simulink model "SingleTrackCANoe"  (R2021b)
settings: Solver=ode1  StartTime=0  StopTime=2  FixedStep=1.0000000000000000e-003  RelTol=1e-3
InitFcn:
  | sampleTime = str2double(get_param(bdroot, 'FixedStep'));
undefined symbols (not defined in the file or in its folder): AccPedalPos, BrakePedalPos, BrakeSwitch, DiscIntNeverNeededParam, DYNA4, EngSpd, IgnitionSwitch, InitialGear, InitialSpeed, IntendedEngTrq, LeftIndicator, MainBrakePress, MaxGear, MDL, MinGear, RefAcc, RefLane, RefLatPos, RefPath, RefPathCurv, RefSpd, RefSpdPreview, RefSpdRetrospect, RightIndicator, SteeringWheelAng, SteeringWheelTrq, UserDefinedRefValue, vm_const
libraries: UtilitiesLibrary x62, simulink x18, WheelSystemModules x14, LongitudinalControllerModules x13, LateralControllerModules x7, AnimationBusselectorModules x5, EnvironmentModules x5, BasicEngineControlModules x5, MiscellaneousControlModules x5, Animation3Modules x4, AuxiliariesModules x4, ReducedTireModules x4
(part 28 of 34)

== system SingleTrackCANoe/SimulationModel/Vehicle/Drivetrain/DrivetrainPhysics/DrivetrainPhysicsInputs/InputFromDrivetrainControlUnit ==
  fromDrivetrainControlUnit : Inport
  TDBusSelector : BusSelector  OutputSignals=TransmissionControlUnit.Gear[-4;20],TransmissionControlUnit.AutomatedManualClutchPos[0_1]
  __TDD__AutomatedManualClutchPos[0_1] : Demux  Outputs=[1]
  __TDD__AutomaticGear[-4;20] : Demux  Outputs=[1]
  AutomaticGear[-4;20]___UNIQUE_1 : Outport  Description=|  PortDimensions=[1]  VectorParamsAs1DForOutWhenUnconnected=off
      | <name>TransmissionControlUnit.Gear[-4;20]</name>
      | <comment></comment>
  AutomatedManualClutchPos[0_1]___UNIQUE_1 : Outport  Description=|  Port=2  PortDimensions=[1]  VectorParamsAs1DForOutWhenUnconnected=off
      | <name>TransmissionControlUnit.AutomatedManualClutchPos[0_1]</name>
      | <comment></comment>
  wires:
  __TDD__AutomatedManualClutchPos[0_1]/1 -> AutomatedManualClutchPos[0_1]___UNIQUE_1/1  "AutomatedManualClutchPos[0_1]"
  __TDD__AutomaticGear[-4;20]/1 -> AutomaticGear[-4;20]___UNIQUE_1/1  "AutomaticGear[-4;20]"
  TDBusSelector/2 -> __TDD__AutomatedManualClutchPos[0_1]/1  "<AutomatedManualClutchPos[0_1]>"
  TDBusSelector/1 -> __TDD__AutomaticGear[-4;20]/1  "<Gear[-4;20]>"
  fromDrivetrainControlUnit/1 -> TDBusSelector/1

== system SingleTrackCANoe/SimulationModel/Vehicle/Drivetrain/DrivetrainPhysics/DrivetrainPhysicsInputs/InputFromEngine ==
  fromEngine : Inport
  TDBusSelector : BusSelector  OutputSignals=EnginePhysics.Mechanics.EngInrt[kg*m**2],EnginePhysics.Mechanics.EngTrq[Nm],EnginePhysics.Mechanics.DerivativeOfEngTrq_wrt_CrankAng[Nm/rad],EnginePhysics.Mechanics.DerivativeOfEngTrq_wrt_EngSpd[Nm/(rad/s)],EnginePhysics.Mechanics.MeanEngFrictionTrq[Nm],EngineControlUnit.EngIdleSpd[rad/s]
  __TDD__DerivativeOfEngTrq_wrt_CrankAng[Nm/rad] : Demux  Outputs=[1]
  __TDD__DerivativeOfEngTrq_wrt_EngSpd[Nm/(rad/s)] : Demux  Outputs=[1]
  __TDD__EngIdleSpd[rad/s] : Demux  Outputs=[1]
  __TDD__EngInrt[kg*m**2] : Demux  Outputs=[1]
  __TDD__EngTrq[Nm] : Demux  Outputs=[1]
  __TDD__MeanEngFrictionTrq[Nm] : Demux  Outputs=[1]
  EngInrt[kg*m**2]___UNIQUE_1 : Outport  Description=|  PortDimensions=[1]  VectorParamsAs1DForOutWhenUnconnected=off
      | <name>EnginePhysics.Mechanics.EngInrt[kg*m**2]</name>
      | <comment></comment>
  EngTrq[Nm]___UNIQUE_1 : Outport  Description=|  Port=2  PortDimensions=[1]  VectorParamsAs1DForOutWhenUnconnected=off
      | <name>EnginePhysics.Mechanics.EngTrq[Nm]</name>
      | <comment></comment>
  DerivativeOfEngTrq_wrt_CrankAng[Nm/rad]___UNIQUE_1 : Outport  Description=|  Port=3  PortDimensions=[1]  VectorParamsAs1DForOutWhenUnconnected=off
      | <name>EnginePhysics.Mechanics.DerivativeOfEngTrq_wrt_CrankAng[Nm/rad]</name>
      | <comment></comment>
  DerivativeOfEngTrq_wrt_EngSpd[Nm/(rad/s)]___UNIQUE_1 : Outport  Description=|  Port=4  PortDimensions=[1]  VectorParamsAs1DForOutWhenUnconnected=off
      | <name>EnginePhysics.Mechanics.DerivativeOfEngTrq_wrt_EngSpd[Nm/(rad/s)]</name>
      | <comment></comment>
  MeanEngFrictionTrq[Nm]___UNIQUE_1 : Outport  Description=|  Port=5  PortDimensions=[1]  VectorParamsAs1DForOutWhenUnconnected=off
      | <name>EnginePhysics.Mechanics.MeanEngFrictionTrq[Nm]</name>
      | <comment></comment>
  EngIdleSpd[rad/s]___UNIQUE_1 : Outport  Description=|  Port=6  PortDimensions=[1]  VectorParamsAs1DForOutWhenUnconnected=off
      | <name>EngineControlUnit.EngIdleSpd[rad/s]</name>
      | <comment></comment>
  wires:
  __TDD__EngIdleSpd[rad/s]/1 -> EngIdleSpd[rad/s]___UNIQUE_1/1  "EngIdleSpd[rad/s]"
  __TDD__MeanEngFrictionTrq[Nm]/1 -> MeanEngFrictionTrq[Nm]___UNIQUE_1/1  "MeanEngFrictionTrq[Nm]"
  __TDD__DerivativeOfEngTrq_wrt_EngSpd[Nm/(rad/s)]/1 -> DerivativeOfEngTrq_wrt_EngSpd[Nm/(rad/s)]___UNIQUE_1/1  "DerivativeOfEngTrq_wrt_EngSpd[Nm/(rad/s)]"
  __TDD__DerivativeOfEngTrq_wrt_CrankAng[Nm/rad]/1 -> DerivativeOfEngTrq_wrt_CrankAng[Nm/rad]___UNIQUE_1/1  "DerivativeOfEngTrq_wrt_CrankAng[Nm/rad]"
  __TDD__EngTrq[Nm]/1 -> EngTrq[Nm]___UNIQUE_1/1  "EngTrq[Nm]"
  __TDD__EngInrt[kg*m**2]/1 -> EngInrt[kg*m**2]___UNIQUE_1/1  "EngInrt[kg*m**2]"
  TDBusSelector/6 -> __TDD__EngIdleSpd[rad/s]/1  "<EngIdleSpd[rad/s]>"
  TDBusSelector/5 -> __TDD__MeanEngFrictionTrq[Nm]/1  "<MeanEngFrictionTrq[Nm]>"
  TDBusSelector/4 -> __TDD__DerivativeOfEngTrq_wrt_EngSpd[Nm/(rad/s)]/1  "<DerivativeOfEngTrq_wrt_EngSpd[Nm/(rad/s)]>"
  TDBusSelector/3 -> __TDD__DerivativeOfEngTrq_wrt_CrankAng[Nm/rad]/1  "<DerivativeOfEngTrq_wrt_CrankAng[Nm/rad]>"
  TDBusSelector/2 -> __TDD__EngTrq[Nm]/1  "<EngTrq[Nm]>"
  TDBusSelector/1 -> __TDD__EngInrt[kg*m**2]/1  "<EngInrt[kg*m**2]>"
  fromEngine/1 -> TDBusSelector/1

== system SingleTrackCANoe/SimulationModel/Vehicle/Drivetrain/DrivetrainPhysics/DrivetrainPhysicsInputs/InputFromWheelSystem ==
  fromWheelSystem : Inport
  TDBusSelector : BusSelector  OutputSignals=FrontLeft.Wheel.RotAcc[rad/s**2],FrontRight.Wheel.RotAcc[rad/s**2],RearLeft.Wheel.RotAcc[rad/s**2],RearRight.Wheel.RotAcc[rad/s**2],FrontLeft.Wheel.RotSpd[rad/s],FrontRight.Wheel.RotSpd[rad/s],RearLeft.Wheel.RotSpd[rad/s],RearRight.Wheel.RotSpd[rad/s],FrontLeft.Wheel.DriveBrakeTrq_wrt_WheelRotAxis(VehSys)[Nm],FrontRight.Wheel.DriveBrakeTrq_wrt_WheelRotAxis(VehSys)[Nm],RearLeft.Wheel.DriveBrakeTrq_wrt_WheelRotAxis(VehSys)[Nm],RearRight.Wheel.DriveBrakeTrq_wrt_WheelRotAxis(VehSys)[Nm],FrontLeft.Wheel.TotalResistanceTorque[Nm],FrontLeft.Wheel.RotAxisInrt[kg*m**2],FrontRight.Wheel.RotAxisInrt[kg*m**2],RearLeft.Wheel.RotAxisInrt[kg*m**2],RearRight.Wheel.RotAxisInrt[kg*m**2],FrontLeft.Wheel.VehBodyReplacementInrt[kg*m**2],FrontLeft.Wheel.KinematicWheelActiveFlag[0;1]
  __TDD__FrontLeft_Wheel_DriveBrakeTrq_wrt_WheelRotAxis(VehSys)[Nm] : Demux  Outputs=[3]
  __TDD__FrontLeft_Wheel_RotAcc[rad/s**2] : Demux  Outputs=1
  __TDD__FrontLeft_Wheel_RotAxisInrt[kg*m**2] : Demux  Outputs=[1]
  __TDD__FrontLeft_Wheel_RotSpd[rad/s] : Demux  Outputs=[1]
  __TDD__FrontRight_Wheel_DriveBrakeTrq_wrt_WheelRotAxis(VehSys)[Nm] : Demux  Outputs=[3]
  __TDD__FrontRight_Wheel_RotAcc[rad/s**2] : Demux  Outputs=1
  __TDD__FrontRight_Wheel_RotAxisInrt[kg*m**2] : Demux  Outputs=[1]
  __TDD__FrontRight_Wheel_RotSpd[rad/s] : Demux  Outputs=[1]
  __TDD__KinematicWheelActiveFlag[0;1] : Demux  Outputs=[1]
  __TDD__RearLeft_Wheel_DriveBrakeTrq_wrt_WheelRotAxis(VehSys)[Nm] : Demux  Outputs=[3]
  __TDD__RearLeft_Wheel_RotAcc[rad/s**2] : Demux  Outputs=1
  __TDD__RearLeft_Wheel_RotAxisInrt[kg*m**2] : Demux  Outputs=[1]
  __TDD__RearLeft_Wheel_RotSpd[rad/s] : Demux  Outputs=[1]
  __TDD__RearRight_Wheel_DriveBrakeTrq_wrt_WheelRotAxis(VehSys)[Nm] : Demux  Outputs=[3]
  __TDD__RearRight_Wheel_RotAcc[rad/s**2] : Demux  Outputs=1
  __TDD__RearRight_Wheel_RotAxisInrt[kg*m**2] : Demux  Outputs=[1]
  __TDD__RearRight_Wheel_RotSpd[rad/s] : Demux  Outputs=[1]
  __TDD__TotalResistanceTorque[Nm] : Demux  Outputs=[1]
  __TDD__VehBodyReplacementInrt[kg*m**2] : Demux  Outputs=[1]
  FrontLeft_Wheel_RotAcc[rad/s**2]___UNIQUE_1 : Outport  Description=|  VectorParamsAs1DForOutWhenUnconnected=off
      | <name>FrontLeft.Wheel.RotAcc[rad/s**2]</name>
      | <comment></comment>
  FrontRight_Wheel_RotAcc[rad/s**2]___UNIQUE_1 : Outport  Description=|  Port=2  VectorParamsAs1DForOutWhenUnconnected=off
      | <name>FrontRight.Wheel.RotAcc[rad/s**2]</name>
      | <comment></comment>
  RearLeft_Wheel_RotAcc[rad/s**2]___UNIQUE_1 : Outport  Description=|  Port=3  VectorParamsAs1DForOutWhenUnconnected=off
      | <name>RearLeft.Wheel.RotAcc[rad/s**2]</name>
      | <comment></comment>
  RearRight_Wheel_RotAcc[rad/s**2]___UNIQUE_1 : Outport  Description=|  Port=4  VectorParamsAs1DForOutWhenUnconnected=off
      | <name>RearRight.Wheel.RotAcc[rad/s**2]</name>
      | <comment></comment>
  FrontLeft_Wheel_RotSpd[rad/s]___UNIQUE_1 : Outport  Description=|  Port=5  PortDimensions=[1]  VectorParamsAs1DForOutWhenUnconnected=off
      | <name>FrontLeft.Wheel.RotSpd[rad/s]</name>
      | <comment></comment>
  FrontRight_Wheel_RotSpd[rad/s]___UNIQUE_1 : Outport  Description=|  Port=6  PortDimensions=[1]  VectorParamsAs1DForOutWhenUnconnected=off
      | <name>FrontRight.Wheel.RotSpd[rad/s]</name>
      | <comment></comment>
  RearLeft_Wheel_RotSpd[rad/s]___UNIQUE_1 : Outport  Description=|  Port=7  PortDimensions=[1]  VectorParamsAs1DForOutWhenUnconnected=off
      | <name>RearLeft.Wheel.RotSpd[rad/s]</name>
      | <comment></comment>
  RearRight_Wheel_RotSpd[rad/s]___UNIQUE_1 : Outport  Description=|  Port=8  PortDimensions=[1]  VectorParamsAs1DForOutWhenUnconnected=off
      | <name>RearRight.Wheel.RotSpd[rad/s]</name>
      | <comment></comment>
  FrontLeft_Wheel_DriveBrakeTrq_wrt_WheelRotAxis(VehSys)[Nm]___UNIQUE_1 : Outport  Description=|  Port=9  PortDimensions=[3]  VectorParamsAs1DForOutWhenUnconnected=off
      | <name>FrontLeft.Wheel.DriveBrakeTrq_wrt_WheelRotAxis(VehSys)[Nm]</name>
      | <comment></comment>
  FrontRight_Wheel_DriveBrakeTrq_wrt_WheelRotAxis(VehSys)[Nm]___UNIQUE_1 : Outport  Description=|  Port=10  PortDimensions=[3]  VectorParamsAs1DForOutWhenUnconnected=off
      | <name>FrontRight.Wheel.DriveBrakeTrq_wrt_WheelRotAxis(VehSys)[Nm]</name>
      | <comment></comment>
  RearLeft_Wheel_DriveBrakeTrq_wrt_WheelRotAxis(VehSys)[Nm]___UNIQUE_1 : Outport  Description=|  Port=11  PortDimensions=[3]  VectorParamsAs1DForOutWhenUnconnected=off
      | <name>RearLeft.Wheel.DriveBrakeTrq_wrt_WheelRotAxis(VehSys)[Nm]</name>
      | <comment></comment>
  RearRight_Wheel_DriveBrakeTrq_wrt_WheelRotAxis(VehSys)[Nm]___UNIQUE_1 : Outport  Description=|  Port=12  PortDimensions=[3]  VectorParamsAs1DForOutWhenUnconnected=off
      | <name>RearRight.Wheel.DriveBrakeTrq_wrt_WheelRotAxis(VehSys)[Nm]</name>
      | <comment></comment>
  TotalResistanceTorque[Nm]___UNIQUE_1 : Outport  Description=|  Port=13  PortDimensions=[1]  VectorParamsAs1DForOutWhenUnconnected=off
      | <name>FrontLeft.Wheel.TotalResistanceTorque[Nm]</name>
      | <comment></comment>
  FrontLeft_Wheel_RotAxisInrt[kg*m**2]___UNIQUE_1 : Outport  Description=|  Port=14  PortDimensions=[1]  VectorParamsAs1DForOutWhenUnconnected=off
      | <name>FrontLeft.Wheel.RotAxisInrt[kg*m**2]</name>
      | <comment></comment>
  FrontRight_Wheel_RotAxisInrt[kg*m**2]___UNIQUE_1 : Outport  Description=|  Port=15  PortDimensions=[1]  VectorParamsAs1DForOutWhenUnconnected=off
      | <name>FrontRight.Wheel.RotAxisInrt[kg*m**2]</name>
      | <comment></comment>
  RearLeft_Wheel_RotAxisInrt[kg*m**2]___UNIQUE_1 : Outport  Description=|  Port=16  PortDimensions=[1]  VectorParamsAs1DForOutWhenUnconnected=off
      | <name>RearLeft.Wheel.RotAxisInrt[kg*m**2]</name>
      | <comment></comment>
  RearRight_Wheel_RotAxisInrt[kg*m**2]___UNIQUE_1 : Outport  Description=|  Port=17  PortDimensions=[1]  VectorParamsAs1DForOutWhenUnconnected=off
      | <name>RearRight.Wheel.RotAxisInrt[kg*m**2]</name>
      | <comment></comment>
  VehBodyReplacementInrt[kg*m**2]___UNIQUE_1 : Outport  Description=|  Port=18  PortDimensions=[1]  VectorParamsAs1DForOutWhenUnconnected=off
      | <name>FrontLeft.Wheel.VehBodyReplacementInrt[kg*m**2]</name>
      | <comment></comment>
  KinematicWheelActiveFlag[0;1]___UNIQUE_1 : Outport  Description=|  Port=19  PortDimensions=[1]  VectorParamsAs1DForOutWhenUnconnected=off
      | <name>FrontLeft.Wheel.KinematicWheelActiveFlag[0;1]</name>
      | <comment></comment>
  wires:
  __TDD__KinematicWheelActiveFlag[0;1]/1 -> KinematicWheelActiveFlag[0;1]___UNIQUE_1/1  "KinematicWheelActiveFlag[0;1]"
  __TDD__VehBodyReplacementInrt[kg*m**2]/1 -> VehBodyReplacementInrt[kg*m**2]___UNIQUE_1/1  "VehBodyReplacementInrt[kg*m**2]"
  __TDD__RearRight_Wheel_RotAxisInrt[kg*m**2]/1 -> RearRight_Wheel_RotAxisInrt[kg*m**2]___UNIQUE_1/1  "RearRight_Wheel_RotAxisInrt[kg*m**2]"
  __TDD__RearLeft_Wheel_RotAxisInrt[kg*m**2]/1 -> RearLeft_Wheel_RotAxisInrt[kg*m**2]___UNIQUE_1/1  "RearLeft_Wheel_RotAxisInrt[kg*m**2]"
  __TDD__FrontRight_Wheel_RotAxisInrt[kg*m**2]/1 -> FrontRight_Wheel_RotAxisInrt[kg*m**2]___UNIQUE_1/1  "FrontRight_Wheel_RotAxisInrt[kg*m**2]"
  __TDD__FrontLeft_Wheel_RotAxisInrt[kg*m**2]/1 -> FrontLeft_Wheel_RotAxisInrt[kg*m**2]___UNIQUE_1/1  "FrontLeft_Wheel_RotAxisInrt[kg*m**2]"
  __TDD__TotalResistanceTorque[Nm]/1 -> TotalResistanceTorque[Nm]___UNIQUE_1/1  "TotalResistanceTorque[Nm]"
  __TDD__RearRight_Wheel_DriveBrakeTrq_wrt_WheelRotAxis(VehSys)[Nm]/1 -> RearRight_Wheel_DriveBrakeTrq_wrt_WheelRotAxis(VehSys)[Nm]___UNIQUE_1/1  "RearRight_Wheel_DriveBrakeTrq_wrt_WheelRotAxis(VehSys)[Nm]"
  __TDD__RearLeft_Wheel_DriveBrakeTrq_wrt_WheelRotAxis(VehSys)[Nm]/1 -> RearLeft_Wheel_DriveBrakeTrq_wrt_WheelRotAxis(VehSys)[Nm]___UNIQUE_1/1  "RearLeft_Wheel_DriveBrakeTrq_wrt_WheelRotAxis(VehSys)[Nm]"
  __TDD__FrontRight_Wheel_DriveBrakeTrq_wrt_WheelRotAxis(VehSys)[Nm]/1 -> FrontRight_Wheel_DriveBrakeTrq_wrt_WheelRotAxis(VehSys)[Nm]___UNIQUE_1/1  "FrontRight_Wheel_DriveBrakeTrq_wrt_WheelRotAxis(VehSys)[Nm]"
  __TDD__FrontLeft_Wheel_DriveBrakeTrq_wrt_WheelRotAxis(VehSys)[Nm]/1 -> FrontLeft_Wheel_DriveBrakeTrq_wrt_WheelRotAxis(VehSys)[Nm]___UNIQUE_1/1  "FrontLeft_Wheel_DriveBrakeTrq_wrt_WheelRotAxis(VehSys)[Nm]"
  __TDD__RearRight_Wheel_RotSpd[rad/s]/1 -> RearRight_Wheel_RotSpd[rad/s]___UNIQUE_1/1  "RearRight_Wheel_RotSpd[rad/s]"
  __TDD__RearLeft_Wheel_RotSpd[rad/s]/1 -> RearLeft_Wheel_RotSpd[rad/s]___UNIQUE_1/1  "RearLeft_Wheel_RotSpd[rad/s]"
  __TDD__FrontRight_Wheel_RotSpd[rad/s]/1 -> FrontRight_Wheel_RotSpd[rad/s]___UNIQUE_1/1  "FrontRight_Wheel_RotSpd[rad/s]"
  __TDD__FrontLeft_Wheel_RotSpd[rad/s]/1 -> FrontLeft_Wheel_RotSpd[rad/s]___UNIQUE_1/1  "FrontLeft_Wheel_RotSpd[rad/s]"
  __TDD__RearRight_Wheel_RotAcc[rad/s**2]/1 -> RearRight_Wheel_RotAcc[rad/s**2]___UNIQUE_1/1  "RearRight_Wheel_RotAcc[rad/s**2]"
  __TDD__RearLeft_Wheel_RotAcc[rad/s**2]/1 -> RearLeft_Wheel_RotAcc[rad/s**2]___UNIQUE_1/1  "RearLeft_Wheel_RotAcc[rad/s**2]"
  __TDD__FrontRight_Wheel_RotAcc[rad/s**2]/1 -> FrontRight_Wheel_RotAcc[rad/s**2]___UNIQUE_1/1  "FrontRight_Wheel_RotAcc[rad/s**2]"
  __TDD__FrontLeft_Wheel_RotAcc[rad/s**2]/1 -> FrontLeft_Wheel_RotAcc[rad/s**2]___UNIQUE_1/1  "FrontLeft_Wheel_RotAcc[rad/s**2]"
  TDBusSelector/19 -> __TDD__KinematicWheelActiveFlag[0;1]/1  "<KinematicWheelActiveFlag[0;1]>"
  TDBusSelector/18 -> __TDD__VehBodyReplacementInrt[kg*m**2]/1  "<VehBodyReplacementInrt[kg*m**2]>"
  TDBusSelector/17 -> __TDD__RearRight_Wheel_RotAxisInrt[kg*m**2]/1  "<RotAxisInrt[kg*m**2]>"
  TDBusSelector/16 -> __TDD__RearLeft_Wheel_RotAxisInrt[kg*m**2]/1  "<RotAxisInrt[kg*m**2]>"
  TDBusSelector/15 -> __TDD__FrontRight_Wheel_RotAxisInrt[kg*m**2]/1  "<RotAxisInrt[kg*m**2]>"
  TDBusSelector/14 -> __TDD__FrontLeft_Wheel_RotAxisInrt[kg*m**2]/1  "<RotAxisInrt[kg*m**2]>"
  TDBusSelector/13 -> __TDD__TotalResistanceTorque[Nm]/1  "<TotalResistanceTorque[Nm]>"
  TDBusSelector/12 -> __TDD__RearRight_Wheel_DriveBrakeTrq_wrt_WheelRotAxis(VehSys)[Nm]/1  "<DriveBrakeTrq_wrt_WheelRotAxis(VehSys)[Nm]>"
  TDBusSelector/11 -> __TDD__RearLeft_Wheel_DriveBrakeTrq_wrt_WheelRotAxis(VehSys)[Nm]/1  "<DriveBrakeTrq_wrt_WheelRotAxis(VehSys)[Nm]>"
  TDBusSelector/10 -> __TDD__FrontRight_Wheel_DriveBrakeTrq_wrt_WheelRotAxis(VehSys)[Nm]/1  "<DriveBrakeTrq_wrt_WheelRotAxis(VehSys)[Nm]>"
  TDBusSelector/9 -> __TDD__FrontLeft_Wheel_DriveBrakeTrq_wrt_WheelRotAxis(VehSys)[Nm]/1  "<DriveBrakeTrq_wrt_WheelRotAxis(VehSys)[Nm]>"
  TDBusSelector/8 -> __TDD__RearRight_Wheel_RotSpd[rad/s]/1  "<RotSpd[rad/s]>"
  TDBusSelector/7 -> __TDD__RearLeft_Wheel_RotSpd[rad/s]/1  "<RotSpd[rad/s]>"
  TDBusSelector/6 -> __TDD__FrontRight_Wheel_RotSpd[rad/s]/1  "<RotSpd[rad/s]>"
  TDBusSelector/5 -> __TDD__FrontLeft_Wheel_RotSpd[rad/s]/1  "<RotSpd[rad/s]>"
  TDBusSelector/4 -> __TDD__RearRight_Wheel_RotAcc[rad/s**2]/1  "<RotAcc[rad/s**2]>"
  TDBusSelector/3 -> __TDD__RearLeft_Wheel_RotAcc[rad/s**2]/1  "<RotAcc[rad/s**2]>"
  TDBusSelector/2 -> __TDD__FrontRight_Wheel_RotAcc[rad/s**2]/1  "<RotAcc[rad/s**2]>"
  TDBusSelector/1 -> __TDD__FrontLeft_Wheel_RotAcc[rad/s**2]/1  "<RotAcc[rad/s**2]>"
  fromWheelSystem/1 -> TDBusSelector/1

== system SingleTrackCANoe/SimulationModel/Vehicle/Drivetrain/DrivetrainPhysics/DrivetrainPhysicsOutputs/ClutchOutput ==
  ClutchStates : Inport
  Bus Selector : BusSelector  OutputSignals=Trq[Nm],ClutchPos[0_1]
  ClutchOutput : Subsystem  Tag=TESIS DYNAware Interface Block  mask{NeedsUpdate=off, SignalInfo=|}
      mask SignalInfo=|
      | {
      |   "Version": "4.6",
      |   "MuxedOutputBusName": "Clutch",
      |   "MuxedInputBusName": "input",
      |   "MuxedInputSelected": false,
      |   "MuxedOutputSelected": true,
      |   "SignalData": [
      |     {
      |       "initialValue": "0.0",
      |       "name": "Trq[Nm]",
      |       "comment": "",
      |       "minString": "",
      |       "maxString": "",
      |       "width": 1,
      |       "dataType": 0,
      |       "signalType": 0,
      |       "createSignal": false,
      |       "outputName": "Trq[Nm]",
      |       "generateSignalAccessBlock": false,
      |       "accessId": "$(parentId).$(blockName).$(outputName)"
      |     },
      |     {
      |       "initialValue": "0.0",
      |       "name": "Pos[0_1]",
      |       "comment": "",
      |       "minString": "",
      |       "maxString": "",
      |       "width": 1,
      |       "dataType": 0,
      |       "signalType": 0,
      |       "createSignal": false,
      |       "outputName": "Pos[0_1]",
      |       "generateSignalAccessBlock": false,
      |       "accessId": "$(parentId).$(blockName).$(outputName)"
      |     }
      |   ]
      | }
      mask prompts: NeedsUpdate "Specify, if subsystem content needs to be updated"; SignalInfo "Signal Info (json)"
      mask help: DYNA4 Interface Block Version 4.6
      mask init:
      | blockName = get_param(gcbh, 'Name');
      | parentId = DYNA4.ModelHandling.AccessID.getFromHierarchy(gcbh);
      | TD.InterfaceBlock.ModelCallbacks.GenerateContent(gcb);
      settings: DeleteFcn=TD.InterfaceBlock.ModelCallbacks.CloseGUI( gcbh );  NameChangeFcn=TD.InterfaceBlock.ModelCallbacks.BlockRenamedHandler(gcbh);  OpenFcn=TD.InterfaceBlock.ModelCallbacks.OpenGUI( gcbh );  CloseFcn=TD.InterfaceBlock.ModelCallbacks.CloseGUI( gcbh );
      mask Display:
      | image('InterfaceBlock.png','center');
      | port_label('input',1, 'Trq[Nm]');
      | port_label('input',2, 'Pos[0_1]');
      | port_label('output',1, 'Clutch');
  Clutch : Outport  VectorParamsAs1DForOutWhenUnconnected=off
  wires:
  Bus Selector/2 -> ClutchOutput/2(Pos[0_1]___UNIQUE_1)  "<ClutchPos[0_1]>"
  Bus Selector/1 -> ClutchOutput/1(Trq[Nm]___UNIQUE_1)  "<Trq[Nm]>"
  ClutchOutput/1(Clutch___UNIQUE_1) -> Clutch/1
  ClutchStates/1 -> Bus Selector/1

== system SingleTrackCANoe/SimulationModel/Vehicle/Drivetrain/DrivetrainPhysics/DrivetrainPhysicsOutputs/DrivetrainPhysicsOutput ==
  EngSpd[rad/s]___UNIQUE_1 : Inport  Description=|  PortDimensions=[1]
      | <name>EngSpd[rad/s]</name>
      | <comment></comment>
  EngAcc[rad/s**2]___UNIQUE_1 : Inport  Description=|  Port=2  PortDimensions=[1]
      | <name>EngAcc[rad/s**2]</name>
      | <comment></comment>
  Clutch___UNIQUE_1 : Inport  Description=|  Port=3
      | <name>Clutch</name>
      | <comment></comment>
  Transmission___UNIQUE_1 : Inport  Description=|  Port=4
      | <name>Transmission</name>
      | <comment></comment>
  TransferCase___UNIQUE_1 : Inport  Description=|  Port=5
      | <name>TransferCase</name>
      | <comment></comment>
  FrontDifferential___UNIQUE_1 : Inport  Description=|  Port=6
      | <name>FrontDifferential</name>
      | <comment></comment>
  FrontLeftShaft___UNIQUE_1 : Inport  Description=|  Port=7
      | <name>FrontLeftShaft</name>
      | <comment></comment>
  FrontRightShaft___UNIQUE_1 : Inport  Description=|  Port=8
      | <name>FrontRightShaft</name>
      | <comment></comment>
  RearDifferential___UNIQUE_1 : Inport  Description=|  Port=9
      | <name>RearDifferential</name>
      | <comment></comment>
  RearLeftShaft___UNIQUE_1 : Inport  Description=|  Port=10
      | <name>RearLeftShaft</name>
      | <comment></comment>
  RearRightShaft___UNIQUE_1 : Inport  Description=|  Port=11
      | <name>RearRightShaft</name>
      | <comment></comment>
  Rear2LeftShaft___UNIQUE_1 : Inport  Description=|  Port=12
      | <name>Rear2LeftShaft</name>
      | <comment></comment>
  Rear2RightShaft___UNIQUE_1 : Inport  Description=|  Port=13
      | <name>Rear2RightShaft</name>
      | <comment></comment>
  Rear3LeftShaft___UNIQUE_1 : Inport  Description=|  Port=14
      | <name>Rear3LeftShaft</name>
      | <comment></comment>
  Rear3RightShaft___UNIQUE_1 : Inport  Description=|  Port=15
      | <name>Rear3RightShaft</name>
      | <comment></comment>
  TotalRatio[-]___UNIQUE_1 : Inport  Description=|  Port=16  PortDimensions=[1]
      | <name>TotalRatio[-]</name>
      | <comment></comment>
  DrivetrainStates___UNIQUE_1 : Inport  Description=|  Port=17
      | <name>DrivetrainStates</name>
      | <comment></comment>
  __TDD__DrivetrainPhysics.EngAcc[rad/s**2] : Demux  Outputs=[1]
  __TDD__DrivetrainPhysics.EngSpd[rad/s] : Demux  Outputs=[1]
  __TDD__DrivetrainPhysics.TotalRatio[-] : Demux  Outputs=[1]
  __TDO__DrivetrainPhysics : BusCreator  Inputs=17
  DrivetrainPhysics___UNIQUE_1 : Outport  Description=|  VectorParamsAs1DForOutWhenUnconnected=off
      | <name>EngSpd[rad/s]</name>
      | <comment></comment>
  wires:
  __TDO__DrivetrainPhysics/1 -> DrivetrainPhysics___UNIQUE_1/1  "DrivetrainPhysics"
  DrivetrainStates___UNIQUE_1/1 -> __TDO__DrivetrainPhysics/17  "DrivetrainStates"
  __TDD__DrivetrainPhysics.TotalRatio[-]/1 -> __TDO__DrivetrainPhysics/16  "TotalRatio[-]"
  TotalRatio[-]___UNIQUE_1/1 -> __TDD__DrivetrainPhysics.TotalRatio[-]/1
  Rear3RightShaft___UNIQUE_1/1 -> __TDO__DrivetrainPhysics/15  "Rear3RightShaft"
  Rear3LeftShaft___UNIQUE_1/1 -> __TDO__DrivetrainPhysics/14  "Rear3LeftShaft"
  Rear2RightShaft___UNIQUE_1/1 -> __TDO__DrivetrainPhysics/13  "Rear2RightShaft"
  Rear2LeftShaft___UNIQUE_1/1 -> __TDO__DrivetrainPhysics/12  "Rear2LeftShaft"
  RearRightShaft___UNIQUE_1/1 -> __TDO__DrivetrainPhysics/11  "RearRightShaft"
  RearLeftShaft___UNIQUE_1/1 -> __TDO__DrivetrainPhysics/10  "RearLeftShaft"
  RearDifferential___UNIQUE_1/1 -> __TDO__DrivetrainPhysics/9  "RearDifferential"
  FrontRightShaft___UNIQUE_1/1 -> __TDO__DrivetrainPhysics/8  "FrontRightShaft"
  FrontLeftShaft___UNIQUE_1/1 -> __TDO__DrivetrainPhysics/7  "FrontLeftShaft"
  FrontDifferential___UNIQUE_1/1 -> __TDO__DrivetrainPhysics/6  "FrontDifferential"
  TransferCase___UNIQUE_1/1 -> __TDO__DrivetrainPhysics/5  "TransferCase"
  Transmission___UNIQUE_1/1 -> __TDO__DrivetrainPhysics/4  "Transmission"
  Clutch___UNIQUE_1/1 -> __TDO__DrivetrainPhysics/3  "Clutch"
  __TDD__DrivetrainPhysics.EngAcc[rad/s**2]/1 -> __TDO__DrivetrainPhysics/2  "EngAcc[rad/s**2]"
  EngAcc[rad/s**2]___UNIQUE_1/1 -> __TDD__DrivetrainPhysics.EngAcc[rad/s**2]/1
  __TDD__DrivetrainPhysics.EngSpd[rad/s]/1 -> __TDO__DrivetrainPhysics/1  "EngSpd[rad/s]"
  EngSpd[rad/s]___UNIQUE_1/1 -> __TDD__DrivetrainPhysics.EngSpd[rad/s]/1

== system SingleTrackCANoe/SimulationModel/Vehicle/Drivetrain/DrivetrainPhysics/DrivetrainPhysicsOutputs/FrontDifferentialOutput ==
  FrontDifferentialStates : Inport
  Bus Selector : BusSelector  OutputSignals=TrqDistributionFactor[0_1]
  FrontDifferentialOutput : Subsystem  Tag=TESIS DYNAware Interface Block  mask{NeedsUpdate=off, SignalInfo=|}
      mask SignalInfo=|
      | {
      |   "Version": "4.6",
      |   "MuxedOutputBusName": "FrontDifferential",
      |   "MuxedInputBusName": "input",
      |   "MuxedInputSelected": false,
      |   "MuxedOutputSelected": true,
      |   "SignalData": {
      |     "initialValue": "0.0",
      |     "name": "TrqDistributionFac[0_1]",
      |     "comment": "",
      |     "minString": "",
      |     "maxString": "",
      |     "width": 1,
      |     "dataType": 0,
      |     "signalType": 0,
      |     "createSignal": false,
      |     "outputName": "TrqDistributionFac[0_1]",
      |     "generateSignalAccessBlock": false,
      |     "accessId": "$(parentId).$(blockName).$(outputName)"
      |   }
      | }
      mask prompts: NeedsUpdate "Specify, if subsystem content needs to be updated"; SignalInfo "Signal Info (json)"
      mask help: DYNA4 Interface Block Version 4.6
      mask init:
      | blockName = get_param(gcbh, 'Name');
      | parentId = DYNA4.ModelHandling.AccessID.getFromHierarchy(gcbh);
      | TD.InterfaceBlock.ModelCallbacks.GenerateContent(gcb);
      settings: DeleteFcn=TD.InterfaceBlock.ModelCallbacks.CloseGUI( gcbh );  NameChangeFcn=TD.InterfaceBlock.ModelCallbacks.BlockRenamedHandler(gcbh);  OpenFcn=TD.InterfaceBlock.ModelCallbacks.OpenGUI( gcbh );  CloseFcn=TD.InterfaceBlock.ModelCallbacks.CloseGUI( gcbh );
      mask Display:
      | image('InterfaceBlock.png','center');
      | port_label('input',1, 'TrqDistributionFac[0_1]');
      | port_label('output',1, 'FrontDifferential');
  FrontDifferential : Outport  VectorParamsAs1DForOutWhenUnconnected=off
  wires:
  FrontDifferentialOutput/1(FrontDifferential___UNIQUE_1) -> FrontDifferential/1
  FrontDifferentialStates/1 -> Bus Selector/1
  Bus Selector/1 -> FrontDifferentialOutput/1(TrqDistributionFac[0_1]___UNIQUE_1)  "<TrqDistributionFactor[0_1]>"

== system SingleTrackCANoe/SimulationModel/Vehicle/Drivetrain/DrivetrainPhysics/DrivetrainPhysicsOutputs/FrontLeftShaftOutput ==
  In1 : Inport
  Bus Selector : BusSelector  OutputSignals=Trq,RotSpd,RotAcc[rad/s**2],DTrq_RotAng,DTrqRotSpd,Inrt[kg*m**2],FrictionTrq[Nm]
  FrontLeftShaftOutput : Subsystem  Tag=TESIS DYNAware Interface Block  mask{NeedsUpdate=off, SignalInfo=|}
      mask SignalInfo=|
      | {
      |   "Version": "4.6",
      |   "MuxedOutputBusName": "FrontLeftShaft",
      |   "MuxedInputBusName": "input",
      |   "MuxedInputSelected": false,
      |   "MuxedOutputSelected": true,
      |   "SignalData": [
      |     {
      |       "initialValue": "0.0",
      |       "name": "Trq[Nm]",
      |       "comment": "",
      |       "minString": "",
      |       "maxString": "",
      |       "width": 1,
      |       "dataType": 0,
      |       "signalType": 0,
      |       "createSignal": false,
      |       "outputName": "Trq[Nm]",
      |       "generateSignalAccessBlock": false,
      |       "accessId": "$(parentId).$(blockName).$(outputName)"
      |     },
      |     {
      |       "initialValue": "0.0",
      |       "name": "RotSpdDifferentialOut[rad/s]",
      |       "comment": "",
      |       "minString": "",
      |       "maxString": "",
      |       "width": 1,
      |       "dataType": 0,
      |       "signalType": 0,
      |       "createSignal": false,
      |       "outputName": "RotSpdDifferentialOut[rad/s]",
      |       "generateSignalAccessBlock": false,
      |       "accessId": "$(parentId).$(blockName).$(outputName)"
      |     },
      |     {
      |       "initialValue": "0.0",
      |       "name": "RotAcc[rad/s**2]",
      |       "comment": "",
      |       "minString": "",
      |       "maxString": "",
      |       "width": 1,
      |       "dataType": 0,
      |       "signalType": 0,
      |       "createSignal": false,
      |       "outputName": "RotAcc[rad/s**2]",
      |       "generateSignalAccessBlock": false,
      |       "accessId": "$(parentId).$(blockName).$(outputName)"
      |     },
      |     {
      |       "initialValue": "0.0",
      |       "name": "DerivativeOfTrq_wrt_RotAng[Nm/rad]",
      |       "comment": "",
      |       "minString": "",
      |       "maxString": "",
      |       "width": 1,
      |       "dataType": 0,
      |       "signalType": 0,
      |       "createSignal": false,
      |       "outputName": "DerivativeOfTrq_wrt_RotAng[Nm/rad]",
      |       "generateSignalAccessBlock": false,
      |       "accessId": "$(parentId).$(blockName).$(outputName)"
      |     },
      |     {
      |       "initialValue": "0.0",
      |       "name": "DerivativeOfTrq_wrt_WheelSpd[Nm/(rad/s)]",
      |       "comment": "",
      |       "minString": "",
      |       "maxString": "",
      |       "width": 1,
      |       "dataType": 0,
      |       "signalType": 0,
      |       "createSignal": false,
      |       "outputName": "DerivativeOfTrq_wrt_WheelSpd[Nm/(rad/s)]",
      |       "generateSignalAccessBlock": false,
      |       "accessId": "$(parentId).$(blockName).$(outputName)"
      |     },
      |     {
      |       "initialValue": "0.0",
      |       "name": "AddInrt[kg*m**2]",
      |       "comment": "",
      |       "minString": "",
      |       "maxString": "",
      |       "width": 1,
      |       "dataType": 0,
      |       "signalType": 0,
      |       "createSignal": false,
      |       "outputName": "AddInrt[kg*m**2]",
      |       "generateSignalAccessBlock": false,
      |       "accessId": "$(parentId).$(blockName).$(outputName)"
      |     },
      |     {
      |       "initialValue": "0.0",
      |       "name": "FrictionTrq[Nm]",
      |       "comment": "",
      |       "minString": "",
      |       "maxString": "",
      |       "width": 1,
      |       "dataType": 0,
      |       "signalType": 0,
      |       "createSignal": false,
      |       "outputName": "FrictionTrq[Nm]",
      |       "generateSignalAccessBlock": false,
      |       "accessId": "$(parentId).$(blockName).$(outputName)"
      |     }
      |   ]
      | }
      mask prompts: NeedsUpdate "Specify, if subsystem content needs to be updated"; SignalInfo "Signal Info (json)"
      mask help: DYNA4 Interface Block Version 4.6
      mask init:
      | blockName = get_param(gcbh, 'Name');
      | parentId = DYNA4.ModelHandling.AccessID.getFromHierarchy(gcbh);
      | TD.InterfaceBlock.ModelCallbacks.GenerateContent(gcb);
      settings: DeleteFcn=TD.InterfaceBlock.ModelCallbacks.CloseGUI( gcbh );  NameChangeFcn=TD.InterfaceBlock.ModelCallbacks.BlockRenamedHandler(gcbh);  OpenFcn=TD.InterfaceBlock.ModelCallbacks.OpenGUI( gcbh );  CloseFcn=TD.InterfaceBlock.ModelCallbacks.CloseGUI( gcbh );
      mask Display:
      | image('InterfaceBlock.png','center');
      | port_label('input',1, 'Trq[Nm]');
      | port_label('input',2, 'RotSpdDifferentialOut[rad/s]');
      | port_label('input',3, 'RotAcc[rad/s**2]');
      | port_label('input',4, 'DerivativeOfTrq_wrt_RotAng[Nm/rad]');
      | port_label('input',5, 'DerivativeOfTrq_wrt_WheelSpd[Nm/(rad/s)]');
      | port_label('input',6, 'AddInrt[kg*m**2]');
      | port_label('input',7, 'FrictionTrq[Nm]');
      | port_label('output',1, 'FrontLeftShaft');
  FrontLeftShaft : Outport  VectorParamsAs1DForOutWhenUnconnected=off
  wires:
  FrontLeftShaftOutput/1(FrontLeftShaft___UNIQUE_1) -> FrontLeftShaft/1
  In1/1 -> Bus Selector/1
  Bus Selector/1 -> FrontLeftShaftOutput/1(Trq[Nm]___UNIQUE_1)  "<Trq>"
  Bus Selector/7 -> FrontLeftShaftOutput/7(FrictionTrq[Nm]___UNIQUE_1)  "<FrictionTrq[Nm]>"
  Bus Selector/6 -> FrontLeftShaftOutput/6(AddInrt[kg*m**2]___UNIQUE_1)  "<Inrt[kg*m**2]>"
  Bus Selector/4 -> FrontLeftShaftOutput/4(DerivativeOfTrq_wrt_RotAng[Nm/rad]___UNIQUE_1)  "<DTrq_RotAng>"
  Bus Selector/5 -> FrontLeftShaftOutput/5(DerivativeOfTrq_wrt_WheelSpd[Nm/(rad/s)]___UNIQUE_1)  "<DTrqRotSpd>"
  Bus Selector/3 -> FrontLeftShaftOutput/3(RotAcc[rad/s**2]___UNIQUE_1)  "<RotAcc[rad/s**2]>"
  Bus Selector/2 -> FrontLeftShaftOutput/2(RotSpdDifferentialOut[rad/s]___UNIQUE_1)  "<RotSpd>"

== system SingleTrackCANoe/SimulationModel/Vehicle/Drivetrain/DrivetrainPhysics/DrivetrainPhysicsOutputs/FrontRightShaftOutput ==
  In1 : Inport
  Bus Selector : BusSelector  OutputSignals=Trq,RotSpd,RotAcc[rad/s**2],DTrqRotAng,DTrqRotSpd,Inrt[kg*m**2],FrictionTrq[Nm]
  FrontRightShaftOutput : Subsystem  Tag=TESIS DYNAware Interface Block  mask{NeedsUpdate=off, SignalInfo=|}
      mask SignalInfo=|
      | {
      |   "Version": "4.6",
      |   "MuxedOutputBusName": "FrontRightShaft",
      |   "MuxedInputBusName": "input",
      |   "MuxedInputSelected": false,
      |   "MuxedOutputSelected": true,
      |   "SignalData": [
      |     {
      |       "initialValue": "0.0",
      |       "name": "Trq[Nm]",
      |       "comment": "",
      |       "minString": "",
      |       "maxString": "",
      |       "width": 1,
      |       "dataType": 0,
      |       "signalType": 0,
      |       "createSignal": false,
      |       "outputName": "Trq[Nm]",
      |       "generateSignalAccessBlock": false,
      |       "accessId": "$(parentId).$(blockName).$(outputName)"
      |     },
      |     {
      |       "initialValue": "0.0",
      |       "name": "RotSpdDifferentialOut[rad/s]",
      |       "comment": "",
      |       "minString": "",
      |       "maxString": "",
      |       "width": 1,
      |       "dataType": 0,
      |       "signalType": 0,
      |       "createSignal": false,
      |       "outputName": "RotSpdDifferentialOut[rad/s]",
      |       "generateSignalAccessBlock": false,
      |       "accessId": "$(parentId).$(blockName).$(outputName)"
      |     },
      |     {
      |       "initialValue": "0.0",
      |       "name": "RotAcc[rad/s**2]",
      |       "comment": "",
      |       "minString": "",
      |       "maxString": "",
      |       "width": 1,
      |       "dataType": 0,
      |       "signalType": 0,
      |       "createSignal": false,
      |       "outputName": "RotAcc[rad/s**2]",
      |       "generateSignalAccessBlock": false,
      |       "accessId": "$(parentId).$(blockName).$(outputName)"
      |     },
      |     {
      |       "initialValue": "0.0",
      |       "name": "DerivativeOfTrq_wrt_RotAng[Nm/rad]",
      |       "comment": "",
      |       "minString": "",
      |       "maxString": "",
      |       "width": 1,
      |       "dataType": 0,
      |       "signalType": 0,
      |       "createSignal": false,
      |       "outputName": "DerivativeOfTrq_wrt_RotAng[Nm/rad]",
      |       "generateSignalAccessBlock": false,
      |       "accessId": "$(parentId).$(blockName).$(outputName)"
      |     },
      |     {
      |       "initialValue": "0.0",
      |       "name": "DerivativeOfTrq_wrt_WheelSpd[Nm/(rad/s)]",
      |       "comment": "",
      |       "minString": "",
      |       "maxString": "",
      |       "width": 1,
      |       "dataType": 0,
      |       "signalType": 0,
      |       "createSignal": false,
      |       "outputName": "DerivativeOfTrq_wrt_WheelSpd[Nm/(rad/s)]",
      |       "generateSignalAccessBlock": false,
      |       "accessId": "$(parentId).$(blockName).$(outputName)"
      |     },
      |     {
      |       "initialValue": "0.0",
      |       "name": "AddInrt[kg*m**2]",
      |       "comment": "",
      |       "minString": "",
      |       "maxString": "",
      |       "width": 1,
      |       "dataType": 0,
      |       "signalType": 0,
      |       "createSignal": false,
      |       "outputName": "AddInrt[kg*m**2]",
      |       "generateSignalAccessBlock": false,
      |       "accessId": "$(parentId).$(blockName).$(outputName)"
      |     },
      |     {
      |       "initialValue": "0.0",
      |       "name": "FrictionTrq[Nm]",
      |       "comment": "",
      |       "minString": "",
      |       "maxString": "",
      |       "width": 1,
      |       "dataType": 0,
      |       "signalType": 0,
      |       "createSignal": false,
      |       "outputName": "FrictionTrq[Nm]",
      |       "generateSignalAccessBlock": false,
      |       "accessId": "$(parentId).$(blockName).$(outputName)"
      |     }
      |   ]
      | }
      mask prompts: NeedsUpdate "Specify, if subsystem content needs to be updated"; SignalInfo "Signal Info (json)"
      mask help: DYNA4 Interface Block Version 4.6
      mask init:
      | blockName = get_param(gcbh, 'Name');
      | parentId = DYNA4.ModelHandling.AccessID.getFromHierarchy(gcbh);
      | TD.InterfaceBlock.ModelCallbacks.GenerateContent(gcb);
      settings: DeleteFcn=TD.InterfaceBlock.ModelCallbacks.CloseGUI( gcbh );  NameChangeFcn=TD.InterfaceBlock.ModelCallbacks.BlockRenamedHandler(gcbh);  OpenFcn=TD.InterfaceBlock.ModelCallbacks.OpenGUI( gcbh );  CloseFcn=TD.InterfaceBlock.ModelCallbacks.CloseGUI( gcbh );
      mask Display:
      | image('InterfaceBlock.png','center');
      | port_label('input',1, 'Trq[Nm]');
      | port_label('input',2, 'RotSpdDifferentialOut[rad/s]');
      | port_label('input',3, 'RotAcc[rad/s**2]');
      | port_label('input',4, 'DerivativeOfTrq_wrt_RotAng[Nm/rad]');
      | port_label('input',5, 'DerivativeOfTrq_wrt_WheelSpd[Nm/(rad/s)]');
      | port_label('input',6, 'AddInrt[kg*m**2]');
      | port_label('input',7, 'FrictionTrq[Nm]');
      | port_label('output',1, 'FrontRightShaft');
  FrontRightShaft : Outport  VectorParamsAs1DForOutWhenUnconnected=off
  wires:
  FrontRightShaftOutput/1(FrontRightShaft___UNIQUE_1) -> FrontRightShaft/1
  Bus Selector/1 -> FrontRightShaftOutput/1(Trq[Nm]___UNIQUE_1)  "<Trq>"
  Bus Selector/7 -> FrontRightShaftOutput/7(FrictionTrq[Nm]___UNIQUE_1)  "<FrictionTrq[Nm]>"
  Bus Selector/6 -> FrontRightShaftOutput/6(AddInrt[kg*m**2]___UNIQUE_1)  "<Inrt[kg*m**2]>"
  Bus Selector/4 -> FrontRightShaftOutput/4(DerivativeOfTrq_wrt_RotAng[Nm/rad]___UNIQUE_1)  "<DTrqRotAng>"
  Bus Selector/5 -> FrontRightShaftOutput/5(DerivativeOfTrq_wrt_WheelSpd[Nm/(rad/s)]___UNIQUE_1)  "<DTrqRotSpd>"
  Bus Selector/3 -> FrontRightShaftOutput/3(RotAcc[rad/s**2]___UNIQUE_1)  "<RotAcc[rad/s**2]>"
  Bus Selector/2 -> FrontRightShaftOutput/2(RotSpdDifferentialOut[rad/s]___UNIQUE_1)  "<RotSpd>"
  In1/1 -> Bus Selector/1

== system SingleTrackCANoe/SimulationModel/Vehicle/Drivetrain/DrivetrainPhysics/DrivetrainPhysicsOutputs/Rear2LeftShaftOutput ==
  __SRC__Rear2LeftShaft.AddInrt[kg*m**2] : Constant  Value=0.0  OutDataTypeStr=Inherit: Inherit via back propagation
  __SRC__Rear2LeftShaft.DerivativeOfTrq_wrt_RotAng[Nm/rad] : Constant  Value=0.0  OutDataTypeStr=Inherit: Inherit via back propagation
  __SRC__Rear2LeftShaft.DerivativeOfTrq_wrt_WheelSpd[Nm/(rad/s)] : Constant  Value=0.0  OutDataTypeStr=Inherit: Inherit via back propagation
  __SRC__Rear2LeftShaft.FrictionTrq[Nm] : Constant  Value=0.0  OutDataTypeStr=Inherit: Inherit via back propagation
  __SRC__Rear2LeftShaft.RotAcc[rad/s**2] : Constant  Value=0.0  OutDataTypeStr=Inherit: Inherit via back propagation
  __SRC__Rear2LeftShaft.RotSpdDifferentialOut[rad/s] : Constant  Value=0.0  OutDataTypeStr=Inherit: Inherit via back propagation
  __SRC__Rear2LeftShaft.Trq[Nm] : Constant  Value=0.0  OutDataTypeStr=Inherit: Inherit via back propagation
  __TDO__Rear2LeftShaft : BusCreator  Inputs=7
  Rear2LeftShaft___UNIQUE_1 : Outport  Description=|  PortDimensions=[7]  VectorParamsAs1DForOutWhenUnconnected=off
      | <name></name>
      | <comment></comment>
  wires:
  __TDO__Rear2LeftShaft/1 -> Rear2LeftShaft___UNIQUE_1/1  "Rear2LeftShaft"
  __SRC__Rear2LeftShaft.FrictionTrq[Nm]/1 -> __TDO__Rear2LeftShaft/7  "FrictionTrq[Nm]"
  __SRC__Rear2LeftShaft.AddInrt[kg*m**2]/1 -> __TDO__Rear2LeftShaft/6  "AddInrt[kg*m**2]"
  __SRC__Rear2LeftShaft.DerivativeOfTrq_wrt_WheelSpd[Nm/(rad/s)]/1 -> __TDO__Rear2LeftShaft/5  "DerivativeOfTrq_wrt_WheelSpd[Nm/(rad/s)]"
  __SRC__Rear2LeftShaft.DerivativeOfTrq_wrt_RotAng[Nm/rad]/1 -> __TDO__Rear2LeftShaft/4  "DerivativeOfTrq_wrt_RotAng[Nm/rad]"
  __SRC__Rear2LeftShaft.RotAcc[rad/s**2]/1 -> __TDO__Rear2LeftShaft/3  "RotAcc[rad/s**2]"
  __SRC__Rear2LeftShaft.RotSpdDifferentialOut[rad/s]/1 -> __TDO__Rear2LeftShaft/2  "RotSpdDifferentialOut[rad/s]"
  __SRC__Rear2LeftShaft.Trq[Nm]/1 -> __TDO__Rear2LeftShaft/1  "Trq[Nm]"

== system SingleTrackCANoe/SimulationModel/Vehicle/Drivetrain/DrivetrainPhysics/DrivetrainPhysicsOutputs/Rear2RightShaftOutput ==
  __SRC__Rear2RightShaft.AddInrt[kg*m**2] : Constant  Value=0.0  OutDataTypeStr=Inherit: Inherit via back propagation
  __SRC__Rear2RightShaft.DerivativeOfTrq_wrt_RotAng[Nm/rad] : Constant  Value=0.0  OutDataTypeStr=Inherit: Inherit via back propagation
  __SRC__Rear2RightShaft.DerivativeOfTrq_wrt_WheelSpd[Nm/(rad/s)] : Constant  Value=0.0  OutDataTypeStr=Inherit: Inherit via back propagation
  __SRC__Rear2RightShaft.FrictionTrq[Nm] : Constant  Value=0.0  OutDataTypeStr=Inherit: Inherit via back propagation
  __SRC__Rear2RightShaft.RotAcc[rad/s**2] : Constant  Value=0.0  OutDataTypeStr=Inherit: Inherit via back propagation
  __SRC__Rear2RightShaft.RotSpdDifferentialOut[rad/s] : Constant  Value=0.0  OutDataTypeStr=Inherit: Inherit via back propagation
  __SRC__Rear2RightShaft.Trq[Nm] : Constant  Value=0.0  OutDataTypeStr=Inherit: Inherit via back propagation
  __TDO__Rear2RightShaft : BusCreator  Inputs=7
  Rear2RightShaft___UNIQUE_1 : Outport  Description=|  PortDimensions=[7]  VectorParamsAs1DForOutWhenUnconnected=off
      | <name></name>
      | <comment></comment>
  wires:
  __TDO__Rear2RightShaft/1 -> Rear2RightShaft___UNIQUE_1/1  "Rear2RightShaft"
  __SRC__Rear2RightShaft.FrictionTrq[Nm]/1 -> __TDO__Rear2RightShaft/7  "FrictionTrq[Nm]"
  __SRC__Rear2RightShaft.AddInrt[kg*m**2]/1 -> __TDO__Rear2RightShaft/6  "AddInrt[kg*m**2]"
  __SRC__Rear2RightShaft.DerivativeOfTrq_wrt_WheelSpd[Nm/(rad/s)]/1 -> __TDO__Rear2RightShaft/5  "DerivativeOfTrq_wrt_WheelSpd[Nm/(rad/s)]"
  __SRC__Rear2RightShaft.DerivativeOfTrq_wrt_RotAng[Nm/rad]/1 -> __TDO__Rear2RightShaft/4  "DerivativeOfTrq_wrt_RotAng[Nm/rad]"
  __SRC__Rear2RightShaft.RotAcc[rad/s**2]/1 -> __TDO__Rear2RightShaft/3  "RotAcc[rad/s**2]"
  __SRC__Rear2RightShaft.RotSpdDifferentialOut[rad/s]/1 -> __TDO__Rear2RightShaft/2  "RotSpdDifferentialOut[rad/s]"
  __SRC__Rear2RightShaft.Trq[Nm]/1 -> __TDO__Rear2RightShaft/1  "Trq[Nm]"

== system SingleTrackCANoe/SimulationModel/Vehicle/Drivetrain/DrivetrainPhysics/DrivetrainPhysicsOutputs/Rear3LeftShaftOutput ==
  __SRC__Rear3LeftShaft.AddInrt[kg*m**2] : Constant  Value=0.0  OutDataTypeStr=Inherit: Inherit via back propagation
  __SRC__Rear3LeftShaft.DerivativeOfTrq_wrt_RotAng[Nm/rad] : Constant  Value=0.0  OutDataTypeStr=Inherit: Inherit via back propagation
  __SRC__Rear3LeftShaft.DerivativeOfTrq_wrt_WheelSpd[Nm/(rad/s)] : Constant  Value=0.0  OutDataTypeStr=Inherit: Inherit via back propagation
  __SRC__Rear3LeftShaft.FrictionTrq[Nm] : Constant  Value=0.0  OutDataTypeStr=Inherit: Inherit via back propagation
  __SRC__Rear3LeftShaft.RotAcc[rad/s**2] : Constant  Value=0.0  OutDataTypeStr=Inherit: Inherit via back propagation
  __SRC__Rear3LeftShaft.RotSpdDifferentialOut[rad/s] : Constant  Value=0.0  OutDataTypeStr=Inherit: Inherit via back propagation
  __SRC__Rear3LeftShaft.Trq[Nm] : Constant  Value=0.0  OutDataTypeStr=Inherit: Inherit via back propagation
  __TDO__Rear3LeftShaft : BusCreator  Inputs=7
  Rear3LeftShaft___UNIQUE_1 : Outport  Description=|  PortDimensions=[7]  VectorParamsAs1DForOutWhenUnconnected=off
      | <name></name>
      | <comment></comment>
  wires:
  __TDO__Rear3LeftShaft/1 -> Rear3LeftShaft___UNIQUE_1/1  "Rear3LeftShaft"
  __SRC__Rear3LeftShaft.FrictionTrq[Nm]/1 -> __TDO__Rear3LeftShaft/7  "FrictionTrq[Nm]"
  __SRC__Rear3LeftShaft.AddInrt[kg*m**2]/1 -> __TDO__Rear3LeftShaft/6  "AddInrt[kg*m**2]"
  __SRC__Rear3LeftShaft.DerivativeOfTrq_wrt_WheelSpd[Nm/(rad/s)]/1 -> __TDO__Rear3LeftShaft/5  "DerivativeOfTrq_wrt_WheelSpd[Nm/(rad/s)]"
  __SRC__Rear3LeftShaft.DerivativeOfTrq_wrt_RotAng[Nm/rad]/1 -> __TDO__Rear3LeftShaft/4  "DerivativeOfTrq_wrt_RotAng[Nm/rad]"
  __SRC__Rear3LeftShaft.RotAcc[rad/s**2]/1 -> __TDO__Rear3LeftShaft/3  "RotAcc[rad/s**2]"
  __SRC__Rear3LeftShaft.RotSpdDifferentialOut[rad/s]/1 -> __TDO__Rear3LeftShaft/2  "RotSpdDifferentialOut[rad/s]"
  __SRC__Rear3LeftShaft.Trq[Nm]/1 -> __TDO__Rear3LeftShaft/1  "Trq[Nm]"

== system SingleTrackCANoe/SimulationModel/Vehicle/Drivetrain/DrivetrainPhysics/DrivetrainPhysicsOutputs/Rear3RightShaftOutput ==
  __SRC__Rear3RightShaft.AddInrt[kg*m**2] : Constant  Value=0.0  OutDataTypeStr=Inherit: Inherit via back propagation
  __SRC__Rear3RightShaft.DerivativeOfTrq_wrt_RotAng[Nm/rad] : Constant  Value=0.0  OutDataTypeStr=Inherit: Inherit via back propagation
  __SRC__Rear3RightShaft.DerivativeOfTrq_wrt_WheelSpd[Nm/(rad/s)] : Constant  Value=0.0  OutDataTypeStr=Inherit: Inherit via back propagation
  __SRC__Rear3RightShaft.FrictionTrq[Nm] : Constant  Value=0.0  OutDataTypeStr=Inherit: Inherit via back propagation
  __SRC__Rear3RightShaft.RotAcc[rad/s**2] : Constant  Value=0.0  OutDataTypeStr=Inherit: Inherit via back propagation
  __SRC__Rear3RightShaft.RotSpdDifferentialOut[rad/s] : Constant  Value=0.0  OutDataTypeStr=Inherit: Inherit via back propagation
  __SRC__Rear3RightShaft.Trq[Nm] : Constant  Value=0.0  OutDataTypeStr=Inherit: Inherit via back propagation
  __TDO__Rear3RightShaft : BusCreator  Inputs=7
  Rear3RightShaft___UNIQUE_1 : Outport  Description=|  PortDimensions=[7]  VectorParamsAs1DForOutWhenUnconnected=off
      | <name></name>
      | <comment></comment>
  wires:
  __TDO__Rear3RightShaft/1 -> Rear3RightShaft___UNIQUE_1/1  "Rear3RightShaft"
  __SRC__Rear3RightShaft.FrictionTrq[Nm]/1 -> __TDO__Rear3RightShaft/7  "FrictionTrq[Nm]"
  __SRC__Rear3RightShaft.AddInrt[kg*m**2]/1 -> __TDO__Rear3RightShaft/6  "AddInrt[kg*m**2]"
  __SRC__Rear3RightShaft.DerivativeOfTrq_wrt_WheelSpd[Nm/(rad/s)]/1 -> __TDO__Rear3RightShaft/5  "DerivativeOfTrq_wrt_WheelSpd[Nm/(rad/s)]"
  __SRC__Rear3RightShaft.DerivativeOfTrq_wrt_RotAng[Nm/rad]/1 -> __TDO__Rear3RightShaft/4  "DerivativeOfTrq_wrt_RotAng[Nm/rad]"
  __SRC__Rear3RightShaft.RotAcc[rad/s**2]/1 -> __TDO__Rear3RightShaft/3  "RotAcc[rad/s**2]"
  __SRC__Rear3RightShaft.RotSpdDifferentialOut[rad/s]/1 -> __TDO__Rear3RightShaft/2  "RotSpdDifferentialOut[rad/s]"
  __SRC__Rear3RightShaft.Trq[Nm]/1 -> __TDO__Rear3RightShaft/1  "Trq[Nm]"

== system SingleTrackCANoe/SimulationModel/Vehicle/Drivetrain/DrivetrainPhysics/DrivetrainPhysicsOutputs/RearDifferentialOutput ==
  RearDifferentialStates : Inport
  Bus Selector : BusSelector  OutputSignals=TrqDistributionFactor[0_1]
  RearDifferentialOutput : Subsystem  Tag=TESIS DYNAware Interface Block  mask{NeedsUpdate=off, SignalInfo=|}
      mask SignalInfo=|
      | {
      |   "Version": "4.6",
      |   "MuxedOutputBusName": "RearDifferential",
      |   "MuxedInputBusName": "input",
      |   "MuxedInputSelected": false,
      |   "MuxedOutputSelected": true,
      |   "SignalData": {
      |     "initialValue": "0.0",
      |     "name": "TrqDistributionFac[0_1]",
      |     "comment": "",
      |     "minString": "",
      |     "maxString": "",
      |     "width": 1,
      |     "dataType": 0,
      |     "signalType": 0,
      |     "createSignal": false,
      |     "outputName": "TrqDistributionFac[0_1]",
      |     "generateSignalAccessBlock": false,
      |     "accessId": "$(parentId).$(blockName).$(outputName)"
      |   }
      | }
      mask prompts: NeedsUpdate "Specify, if subsystem content needs to be updated"; SignalInfo "Signal Info (json)"
      mask help: DYNA4 Interface Block Version 4.6
      mask init:
      | blockName = get_param(gcbh, 'Name');
      | parentId = DYNA4.ModelHandling.AccessID.getFromHierarchy(gcbh);
      | TD.InterfaceBlock.ModelCallbacks.GenerateContent(gcb);
      settings: DeleteFcn=TD.InterfaceBlock.ModelCallbacks.CloseGUI( gcbh );  NameChangeFcn=TD.InterfaceBlock.ModelCallbacks.BlockRenamedHandler(gcbh);  OpenFcn=TD.InterfaceBlock.ModelCallbacks.OpenGUI( gcbh );  CloseFcn=TD.InterfaceBlock.ModelCallbacks.CloseGUI( gcbh );
      mask Display:
      | image('InterfaceBlock.png','center');
      | port_label('input',1, 'TrqDistributionFac[0_1]');
      | port_label('output',1, 'RearDifferential');
  RearDifferential : Outport  VectorParamsAs1DForOutWhenUnconnected=off
  wires:
  Bus Selector/1 -> RearDifferentialOutput/1(TrqDistributionFac[0_1]___UNIQUE_1)  "<TrqDistributionFactor[0_1]>"
  RearDifferentialStates/1 -> Bus Selector/1
  RearDifferentialOutput/1(RearDifferential___UNIQUE_1) -> RearDifferential/1
